simulink model "heat_exchanger"  (R2017b)
settings: Solver=VariableStepAuto  StartTime=0.0  StopTime=100  RelTol=1e-3
model workspace: external: MAT-File C:\Users\Alexander\Google Drive\Chalmers\Master Thesis\Matlab_Simulink\heat_exchanger_config.mat (data not in the file)
values from neighbouring files (symbols this model uses):
  B = [(cp_H2O*(T_H2O_in - x_H2O_0))/(m_H2O*cp_H2O) -(cp_wort*(T_wort_in - x_wort_0))/(m_wort*cp_wort) ... (first row only)    [heat_exchanger_config.m]
  C = Kc * (1 + 1/(tauc*s))    [Heat_test.m]    (also in heat_exchanger_config.m = [1 0 ; 0 1])
  cp_wort = 4000    [heat_exchanger_config.m]
  D = zeros(length(C(:,1)),length(B(1,:)))    [heat_exchanger_config.m]
  HE_delay = 5    [heat_exchanger_config.m]
  Kr = inv(D-(C-D*LQR_gain)*inv(A-B*LQR_gain))    [heat_exchanger_config.m]
  Reference = [25 0]    [heat_exchanger_config.m]
  rho_wort = 1.06    [heat_exchanger_config.m]
  T_H2O_in = 10    [heat_exchanger_config.m]
  T_wort_in = 70    [heat_exchanger_config.m]
  water_low_lim = 0.1    [heat_exchanger_config.m]
  water_up_lim = 10    [heat_exchanger_config.m]
  wort_low_lim = 0.1    [heat_exchanger_config.m]
  wort_up_lim = 10    [heat_exchanger_config.m]
undefined symbols (not defined in the file or in its folder): A, LQR_gain
settings Model: PauseTimes=0  Creator=Alexander  LastModifiedBy=Alexander

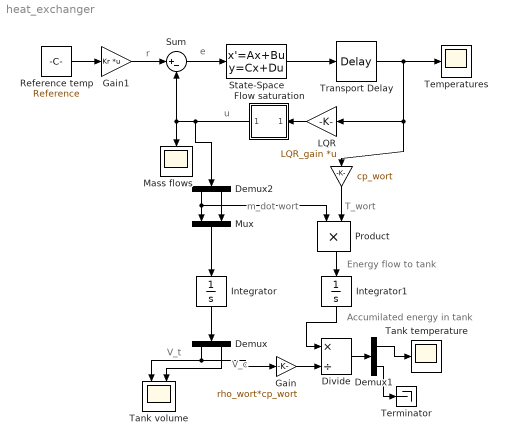
== system heat_exchanger ==
  note: Accumilated energy in tank
  note: Energy flow to tank
  note: T_wort
  note: m_dot wort
  note: V_c
  note: V_t
  note: r
  note: u
  note: e
  " " : Gain  Gain=cp_wort
  Demux : Demux  Outputs=2
  Demux1 : Demux  Outputs=2
  Demux2 : Demux  Outputs=2
  Divide : Product  Inputs=*/
  Flow saturation : Subsystem
  Gain : Gain  Gain=rho_wort*cp_wort
  Gain1 : Gain  Gain=Kr  Multiplication=Matrix(K*u) (u vector)
  Integrator : Integrator
  Integrator1 : Integrator
  LQR : Gain  Gain=LQR_gain  Multiplication=Matrix(K*u) (u vector)
  Mass flows : Scope
  Mux : Mux  Inputs=2
  Product : Product
  Reference temp : Constant  Value=Reference
  State-Space : StateSpace  A=A  B=B  C=C  D=D  InitialCondition=[T_wort_in T_H2O_in]
  Sum : Sum  Inputs=|+-
  Tank temperature : Scope
  Tank volume : Scope  NumInputPorts=2
  Temperatures : Scope
  Terminator : Terminator
  Transport Delay : TransportDelay  DelayTime=HE_delay
  wires:
  Sum/1 -> State-Space/1
  Reference temp/1 -> Gain1/1
  Integrator/1 -> Demux/1
  Demux/1 -> Tank volume/1, Gain/1
  Demux/2 -> Tank volume/2
  Mux/1 -> Integrator/1
  Demux2/1 -> Product/1, Mux/1
  Demux2/2 -> Mux/2
  Product/1 -> Integrator1/1
  " "/1 -> Product/2
  Integrator1/1 -> Divide/1
  Gain/1 -> Divide/2
  Gain1/1 -> Sum/1
  LQR/1 -> Flow saturation/1(In1)
  State-Space/1 -> Transport Delay/1
  Transport Delay/1 -> LQR/1, " "/1, Temperatures/1
  Divide/1 -> Demux1/1
  Demux1/1 -> Tank temperature/1
  Demux1/2 -> Terminator/1
  Flow saturation/1(Out1) -> Demux2/1, Sum/2, Mass flows/1

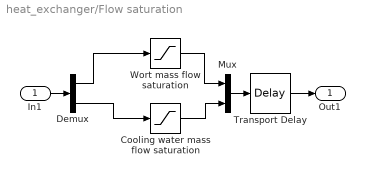
== system heat_exchanger/Flow saturation ==
  In1 : Inport
  Cooling water mass flow saturation : Saturate  UpperLimit=water_up_lim  LowerLimit=water_low_lim
  Demux : Demux  Outputs=2
  Mux : Mux  Inputs=2
  Transport Delay : TransportDelay  DelayTime=HE_delay
  "Wort mass flow saturation " : Saturate  UpperLimit=wort_up_lim  LowerLimit=wort_low_lim
  Out1 : Outport
  wires:
  In1/1 -> Demux/1
  Demux/1 -> "Wort mass flow saturation "/1
  Demux/2 -> Cooling water mass flow saturation/1
  Mux/1 -> Transport Delay/1
  "Wort mass flow saturation "/1 -> Mux/1
  Cooling water mass flow saturation/1 -> Mux/2
  Transport Delay/1 -> Out1/1
